simulink model "simulare_redresor"  (R2020b)
settings: Solver=VariableStepAuto  StartTime=0.0  StopTime=1  RelTol=1e-3
values from neighbouring files (symbols this model uses):
  Cf = 48.76/1000    (= 0.04876)    [simulare.m]
  Ki = 1/Rrt1/Cf    (= 77.6253354191)    [simulare.m]
  Rs = 2.66    [iraep.m]    (also in simulare.m)
  U021Max = U021 * sqrt(2)    [simulare.m]
settings Model: Creator=drago  LastModifiedBy=Alex

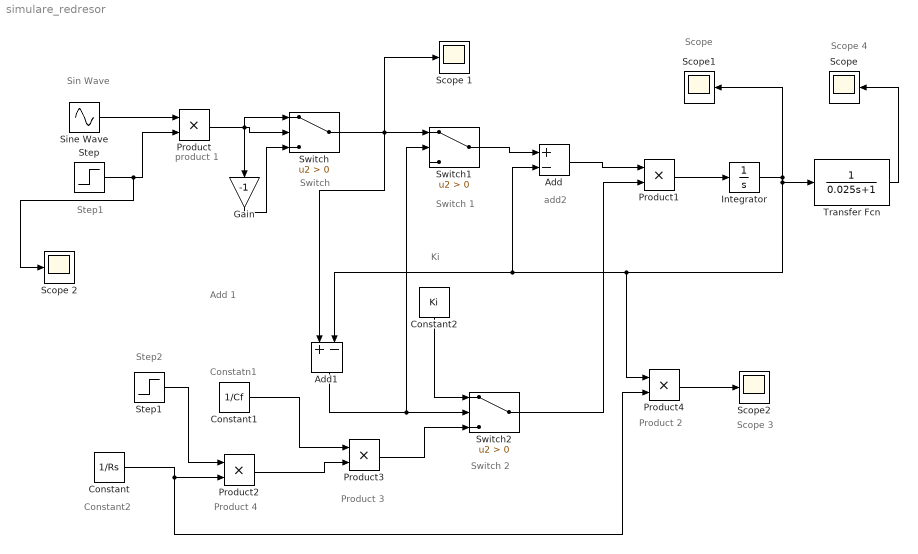
== system simulare_redresor ==
  note: Sin Wave
  note: Scope 3
  note: add2
  note: Switch 2
  note: Product 2
  note: Scope
  note: Switch 1
  note: Add 1
  note: product 1
  note: Product 4
  note: Product 3
  note: Step1
  note: Constatn1
  note: Scope 4
  note: Constant2
  note: Ki
  note: Step2
  note: Switch
  Add : Sum  Inputs=+-
  Add1 : Sum  Inputs=+-
  Constant : Constant  Value=1/Rs
  Constant1 : Constant  Value=1/Cf
  Constant2 : Constant  Value=Ki
  Gain : Gain  Gain=-1
  Integrator : Integrator
  Product{,1..4} (5 alike) : Product
  Scope : Scope
  Scope 1 : Scope
  Scope 2 : Scope
  Scope1 : Scope
  Scope2 : Scope
  Sine Wave : Sin  Amplitude=U021Max  Frequency=314  SampleTime=0
  Step : Step  Time=2  Before=1  After=0.85  SampleTime=0
  Step1 : Step  SampleTime=0
  Switch : Switch  Criteria=u2 > Threshold
  Switch1 : Switch  Criteria=u2 > Threshold
  Switch2 : Switch  Criteria=u2 > Threshold
  Transfer Fcn : TransferFcn  Denominator=[0.025 1]
  wires:
  Product4/1 -> Scope2/1
  Integrator/1 -> Transfer Fcn/1, Product4/1, Add/2, Add1/2, Scope1/1
  Product1/1 -> Integrator/1
  Switch/1 -> Add1/1, Switch1/1, Scope 1/1
  Transfer Fcn/1 -> Scope/1
  Gain/1 -> Switch/3
  Product/1 -> Switch/1, Switch/2, Gain/1
  Step/1 -> Scope 2/1, Product/2
  Sine Wave/1 -> Product/1
  Product3/1 -> Switch2/3
  Add/1 -> Product1/1
  Constant2/1 -> Switch2/1
  Product2/1 -> Product3/2
  Constant/1 -> Product4/2, Product2/2
  Switch1/1 -> Add/1
  Step1/1 -> Product2/1
  Constant1/1 -> Product3/1
  Add1/1 -> Switch1/2, Switch2/2
  Switch2/1 -> Product1/2
